simulink model "statefdbk"  (R2023a)
settings: Solver=VariableStepAuto  StartTime=0.0  StopTime=10.0  RelTol=1e-3
values from neighbouring files (symbols this model uses):
  K = lqr(A,B,Qr,Rr)    [Homework1.m]    (also in Main.m = lqr(A, B, Qr, Rr); Question9_Experiments.m = lqr(A, B, Qr, Rr); simulater.m = lqr(A, B, Qr, Rr))
settings Model: Creator=joaodias  LastModifiedBy=joaodias

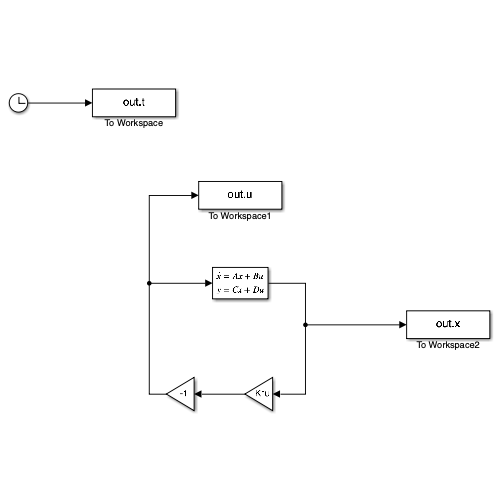
[thumbnail: Simulink's stored preview of the top-level diagram]
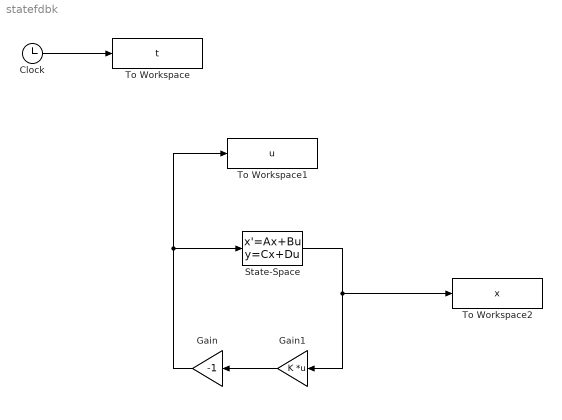
== system statefdbk ==
  Clock : Clock
  Gain : Gain  Gain=-1
  Gain1 : Gain  Gain=K  Multiplication=Matrix(K*u)
  State-Space : StateSpace  InitialCondition=0
  To Workspace : ToWorkspace  VariableName=t  SaveFormat=Timeseries  SampleTime=-1
  To Workspace1 : ToWorkspace  VariableName=u  SaveFormat=Timeseries  SampleTime=-1
  To Workspace2 : ToWorkspace  VariableName=x  SaveFormat=Timeseries  SampleTime=-1
  wires:
  Clock/1 -> To Workspace/1
  State-Space/1 -> To Workspace2/1, Gain1/1
  Gain1/1 -> Gain/1
  Gain/1 -> State-Space/1, To Workspace1/1
